simulink model "roach2_fengine_nlb"  (R2013b)
settings: Solver=VariableStepDiscrete  SolverMode=SingleTasking  StartTime=0.0  StopTime=10.0  RelTol=1e-3
undefined symbols (not defined in the file or in its folder): sfp
libraries: xbsIndex_r4 x3316, xps_library x74, casper_library_sources x16, casper_library_misc x7
(part 16 of 38)

== system roach2_fengine_nlb/eth/3/gbe_gpu_en ==
  in : Inport
  Logical : xbsIndex_r4/Logical  logical_function=AND  inputs=2  en=off  latency=1  precision=Full  arith_type=Unsigned  n_bits=16  bin_pt=0  align_bp=on  dbl_ovrd=off  block_type=logical
  out : Outport
  wires:
  [gbe_gpu_en] -> Logical/1
  Logical/1 -> out/1
  in/1 -> Logical/2

== system roach2_fengine_nlb/eth/3/gbe_sw_en ==
  in : Inport
  Logical : xbsIndex_r4/Logical  logical_function=AND  inputs=2  en=off  latency=0  precision=Full  arith_type=Unsigned  n_bits=16  bin_pt=0  align_bp=on  dbl_ovrd=off  block_type=logical
  out : Outport
  wires:
  in/1 -> Logical/2
  Logical/1 -> out/1
  [gbe_sw_en] -> Logical/1

== system roach2_fengine_nlb/eth/3/gpu_mon ==
  oflow : Inport
  Counter3 : xbsIndex_r4/Counter  cnt_type=Free Running  cnt_to=Inf  operation=Up  start_count=0  cnt_by_val=1  arith_type=Unsigned  n_bits=32  bin_pt=0  load_pin=off  rst=on  en=on  explicit_period=on  period=1  dbl_ovrd=off  use_behavioral_HDL=off  implementation=Fabric  block_type=counter
  Delay3 : xbsIndex_r4/Delay  rst=off  infoeditControl=Selection of Reset will increase slice count due to use of real FFs and instead of SRLs  en=off  latency=1  dbl_ovrd=off  reg_retiming=off  block_type=delay
  Delay6 : xbsIndex_r4/Delay  rst=off  infoeditControl=Selection of Reset will increase slice count due to use of real FFs and instead of SRLs  en=off  latency=1  dbl_ovrd=off  reg_retiming=off  block_type=delay
  oflow_cnt : Outport
  wires:
  Delay3/1 -> Counter3/2
  oflow/1 -> Delay3/1
  Delay6/1 -> oflow_cnt/1
  [cnt_rst] -> Counter3/1
  Counter3/1 -> Delay6/1

== system roach2_fengine_nlb/eth/3/sw_mon ==
  bfr : Inport
  orun : Inport  Port=2
  oflow : Inport  Port=3
  Counter1 : xbsIndex_r4/Counter  cnt_type=Free Running  cnt_to=Inf  operation=Up  start_count=0  cnt_by_val=1  arith_type=Unsigned  n_bits=32  bin_pt=0  load_pin=off  rst=on  en=on  explicit_period=on  period=1  dbl_ovrd=off  use_behavioral_HDL=off  implementation=Fabric  block_type=counter
  Counter2 : xbsIndex_r4/Counter  cnt_type=Free Running  cnt_to=Inf  operation=Up  start_count=0  cnt_by_val=1  arith_type=Unsigned  n_bits=32  bin_pt=0  load_pin=off  rst=on  en=on  explicit_period=on  period=1  dbl_ovrd=off  use_behavioral_HDL=off  implementation=Fabric  block_type=counter
  Counter3 : xbsIndex_r4/Counter  cnt_type=Free Running  cnt_to=Inf  operation=Up  start_count=0  cnt_by_val=1  arith_type=Unsigned  n_bits=32  bin_pt=0  load_pin=off  rst=on  en=on  explicit_period=on  period=1  dbl_ovrd=off  use_behavioral_HDL=off  implementation=Fabric  block_type=counter
  Delay{1..3,5..7} (6 alike) : xbsIndex_r4/Delay  rst=off  infoeditControl=Selection of Reset will increase slice count due to use of real FFs and instead of SRLs  en=off  latency=1  dbl_ovrd=off  reg_retiming=off  block_type=delay
  bfr_cnt : Outport
  orun_cnt : Outport  Port=2
  oflow_cnt : Outport  Port=3
  wires:
  Counter2/1 -> Delay5/1
  [cnt_rst] -> Counter2/1
  Counter1/1 -> Delay7/1
  [cnt_rst] -> Counter1/1
  Counter3/1 -> Delay6/1
  [cnt_rst] -> Counter3/1
  Delay5/1 -> bfr_cnt/1
  bfr/1 -> Delay1/1
  Delay7/1 -> orun_cnt/1
  orun/1 -> Delay2/1
  Delay6/1 -> oflow_cnt/1
  oflow/1 -> Delay3/1
  Delay1/1 -> Counter2/2
  Delay2/1 -> Counter1/2
  Delay3/1 -> Counter3/2

== system roach2_fengine_nlb/input/mux_0_31/in_snap ==
  In1 : Inport
  In2 : Inport  Port=2
  In3 : Inport  Port=3
  In4 : Inport  Port=4
  BitBasher : xbsIndex_r4/BitBasher  bitexpr=|  display_expr=off  sr_1=1  arith_type1=Unsigned  bin_pt1=0  sr_2=2  arith_type2=Unsigned  bin_pt2=0  sr_3=3  arith_type3=Unsigned  bin_pt3=0  sr_4=4  arith_type4=Unsigned  bin_pt4=0  dbl_ovrd=off  block_type=bitbasher
      | <!DOCTYPE HTML PUBLIC "-//W3C//DTD HTML 4.0//EN" "http://www.w3.org/TR/REC-html40/strict.dtd">
      | <html><head><meta name="qrichtext" content="1" /><style type="text/css">
      | p, li { white-space: pre-wrap; }
      | </style></head><body style=" font-family:'Sans'; font-size:10pt; font-weight:400; font-style:normal;">
      | <p style=" margin-top:12px; margin-bottom:12px; margin-left:0px; margin-right:0px; -qt-block-indent:0; text-indent:0px;"><span style=" font-family:'MS Shell Dlg'; font-size:8pt;">w32={d8,c8,b8,a8}</span></p></body></html>
  Delay : xbsIndex_r4/Delay  rst=off  infoeditControl=Selection of Reset will increase slice count due to use of real FFs and instead of SRLs  en=off  latency=3  dbl_ovrd=off  reg_retiming=on  block_type=delay
  tag scope: in_snap=global
  wires:
  BitBasher/1 -> Delay/1
  Delay/1 -> [in_snap]
  In1/1 -> BitBasher/1
  In2/1 -> BitBasher/2
  In3/1 -> BitBasher/3
  In4/1 -> BitBasher/4

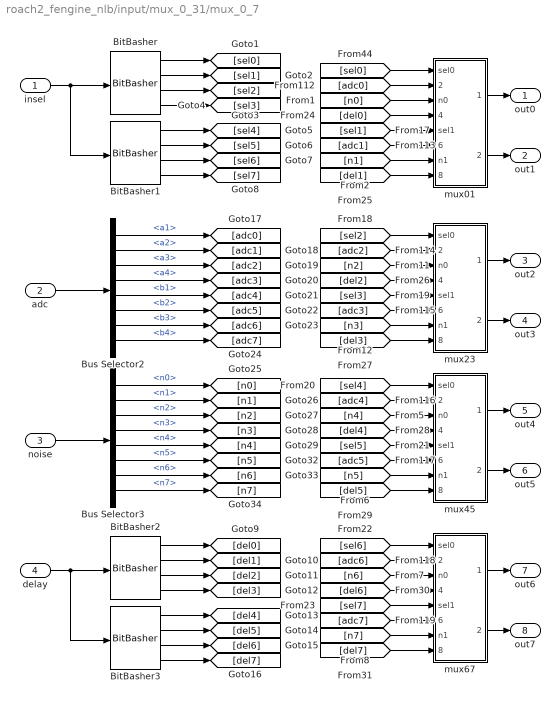
== system roach2_fengine_nlb/input/mux_0_31/mux_0_7 ==
  insel : Inport
  adc : Inport  Port=2
  noise : Inport  Port=3
  delay : Inport  Port=4
  BitBasher : xbsIndex_r4/BitBasher  bitexpr=|  display_expr=off  sr_1=1  arith_type1=Unsigned  bin_pt1=0  sr_2=2  arith_type2=Unsigned  bin_pt2=0  sr_3=3  arith_type3=Unsigned  bin_pt3=0  sr_4=4  arith_type4=Unsigned  bin_pt4=0  dbl_ovrd=off  block_type=bitbasher
      | <!DOCTYPE HTML PUBLIC "-//W3C//DTD HTML 4.0//EN" "http://www.w3.org/TR/REC-html40/strict.dtd">
      | <html><head><meta name="qrichtext" content="1" /><style type="text/css">
      | p, li { white-space: pre-wrap; }
      | </style></head><body style=" font-family:'Sans'; font-size:10pt; font-weight:400; font-style:normal;">
      | <p style=" margin-top:12px; margin-bottom:12px; margin-left:0px; margin-right:0px; -qt-block-indent:0; text-indent:0px;"><span style=" font-family:'MS Shell Dlg'; font-size:8pt;">s0={sel[1:0]}<br />s1={sel[5:4]}<br />s2={sel[9:8]}<br />s3={sel[13:12]}</span></p></body></html>
  BitBasher1 : xbsIndex_r4/BitBasher  bitexpr=|  display_expr=off  sr_1=1  arith_type1=Unsigned  bin_pt1=0  sr_2=2  arith_type2=Unsigned  bin_pt2=0  sr_3=3  arith_type3=Unsigned  bin_pt3=0  sr_4=4  arith_type4=Unsigned  bin_pt4=0  dbl_ovrd=off  block_type=bitbasher
      | <!DOCTYPE HTML PUBLIC "-//W3C//DTD HTML 4.0//EN" "http://www.w3.org/TR/REC-html40/strict.dtd">
      | <html><head><meta name="qrichtext" content="1" /><style type="text/css">
      | p, li { white-space: pre-wrap; }
      | </style></head><body style=" font-family:'Sans'; font-size:10pt; font-weight:400; font-style:normal;">
      | <p style=" margin-top:12px; margin-bottom:12px; margin-left:0px; margin-right:0px; -qt-block-indent:0; text-indent:0px;"><span style=" font-family:'MS Shell Dlg'; font-size:8pt;">s4={sel[17:16]}<br />s5={sel[21:20]}<br />s6={sel[25:24]}<br />s7={sel[29:28]}</span></p></body></html>
  BitBasher2 : xbsIndex_r4/BitBasher  bitexpr=|  display_expr=off  sr_1=1  arith_type1=Unsigned  bin_pt1=0  sr_2=2  arith_type2=Unsigned  bin_pt2=0  sr_3=3  arith_type3=Unsigned  bin_pt3=0  sr_4=4  arith_type4=Unsigned  bin_pt4=0  dbl_ovrd=off  block_type=bitbasher
      | <!DOCTYPE HTML PUBLIC "-//W3C//DTD HTML 4.0//EN" "http://www.w3.org/TR/REC-html40/strict.dtd">
      | <html><head><meta name="qrichtext" content="1" /><style type="text/css">
      | p, li { white-space: pre-wrap; }
      | </style></head><body style=" font-family:'Sans'; font-size:10pt; font-weight:400; font-style:normal;">
      | <p style=" margin-top:12px; margin-bottom:12px; margin-left:0px; margin-right:0px; -qt-block-indent:0; text-indent:0px;"><span style=" font-family:'MS Shell Dlg'; font-size:8pt;">d0={delay[7:0]}<br />d1={delay[15:8]}<br />d2={delay[23:16]}<br />d3={delay[31:24]}</span></p></body></html>
  BitBasher3 : xbsIndex_r4/BitBasher  bitexpr=|  display_expr=off  sr_1=1  arith_type1=Unsigned  bin_pt1=0  sr_2=2  arith_type2=Unsigned  bin_pt2=0  sr_3=3  arith_type3=Unsigned  bin_pt3=0  sr_4=4  arith_type4=Unsigned  bin_pt4=0  dbl_ovrd=off  block_type=bitbasher
      | <!DOCTYPE HTML PUBLIC "-//W3C//DTD HTML 4.0//EN" "http://www.w3.org/TR/REC-html40/strict.dtd">
      | <html><head><meta name="qrichtext" content="1" /><style type="text/css">
      | p, li { white-space: pre-wrap; }
      | </style></head><body style=" font-family:'Sans'; font-size:10pt; font-weight:400; font-style:normal;">
      | <p style=" margin-top:12px; margin-bottom:12px; margin-left:0px; margin-right:0px; -qt-block-indent:0; text-indent:0px;"><span style=" font-family:'MS Shell Dlg'; font-size:8pt;">d4={delay[39:32]}<br />d5={delay[47:40]}<br />d6={delay[55:48]}<br />d7={delay[63:56]}</span></p></body></html>
  Bus Selector2 : BusSelector  OutputSignals=a1,a2,a3,a4,b1,b2,b3,b4
  Bus Selector3 : BusSelector  OutputSignals=n0,n1,n2,n3,n4,n5,n6,n7
  mux01 : Subsystem
  mux23 : Subsystem
  mux45 : Subsystem
  mux67 : Subsystem
  out0 : Outport
  out1 : Outport  Port=2
  out2 : Outport  Port=3
  out3 : Outport  Port=4
  out4 : Outport  Port=5
  out5 : Outport  Port=6
  out6 : Outport  Port=7
  out7 : Outport  Port=8
  wires:
  [sel0] -> mux01/1(sel0)
  [adc0] -> mux01/2(adc0)
  [del0] -> mux01/4(delay0)
  [sel1] -> mux01/5(sel1)
  [adc1] -> mux01/6(adc1)
  [del1] -> mux01/8(delay1)
  BitBasher/1 -> [sel0]
  BitBasher/2 -> [sel1]
  BitBasher/3 -> [sel2]
  BitBasher/4 -> [sel3]
  BitBasher1/1 -> [sel4]
  BitBasher1/2 -> [sel5]
  BitBasher1/3 -> [sel6]
  BitBasher1/4 -> [sel7]
  [n0] -> mux01/3(n0)
  [n1] -> mux01/7(n1)
  [sel2] -> mux23/1(sel0)
  [adc2] -> mux23/2(adc0)
  [n2] -> mux23/3(n0)
  [del2] -> mux23/4(delay0)
  [sel3] -> mux23/5(sel1)
  [adc3] -> mux23/6(adc1)
  [n3] -> mux23/7(n1)
  [del3] -> mux23/8(delay1)
  [sel4] -> mux45/1(sel0)
  [adc4] -> mux45/2(adc0)
  [n4] -> mux45/3(n0)
  [del4] -> mux45/4(delay0)
  [sel5] -> mux45/5(sel1)
  [adc5] -> mux45/6(adc1)
  [n5] -> mux45/7(n1)
  [del5] -> mux45/8(delay1)
  [sel6] -> mux67/1(sel0)
  [adc6] -> mux67/2(adc0)
  [n6] -> mux67/3(n0)
  [del6] -> mux67/4(delay0)
  [sel7] -> mux67/5(sel1)
  [adc7] -> mux67/6(adc1)
  [n7] -> mux67/7(n1)
  [del7] -> mux67/8(delay1)
  insel/1 -> BitBasher1/1, BitBasher/1
  BitBasher2/1 -> [del0]
  BitBasher2/2 -> [del1]
  BitBasher2/3 -> [del2]
  BitBasher2/4 -> [del3]
  BitBasher3/1 -> [del4]
  BitBasher3/2 -> [del5]
  BitBasher3/3 -> [del6]
  BitBasher3/4 -> [del7]
  delay/1 -> BitBasher3/1, BitBasher2/1
  Bus Selector2/1 -> [adc0]  "<a1>"
  Bus Selector2/2 -> [adc1]  "<a2>"
  Bus Selector2/3 -> [adc2]  "<a3>"
  Bus Selector2/4 -> [adc3]  "<a4>"
  Bus Selector2/5 -> [adc4]  "<b1>"
  Bus Selector2/6 -> [adc5]  "<b2>"
  Bus Selector2/7 -> [adc6]  "<b3>"
  Bus Selector2/8 -> [adc7]  "<b4>"
  Bus Selector3/1 -> [n0]  "<n0>"
  Bus Selector3/2 -> [n1]  "<n1>"
  Bus Selector3/3 -> [n2]  "<n2>"
  Bus Selector3/4 -> [n3]  "<n3>"
  Bus Selector3/5 -> [n4]  "<n4>"
  Bus Selector3/6 -> [n5]  "<n5>"
  Bus Selector3/7 -> [n6]  "<n6>"
  Bus Selector3/8 -> [n7]  "<n7>"
  mux01/1(out0) -> out0/1
  mux01/2(out1) -> out1/1
  mux23/1(out0) -> out2/1
  adc/1 -> Bus Selector2/1
  mux23/2(out1) -> out3/1
  mux45/1(out0) -> out4/1
  noise/1 -> Bus Selector3/1
  mux45/2(out1) -> out5/1
  mux67/1(out0) -> out6/1
  mux67/2(out1) -> out7/1

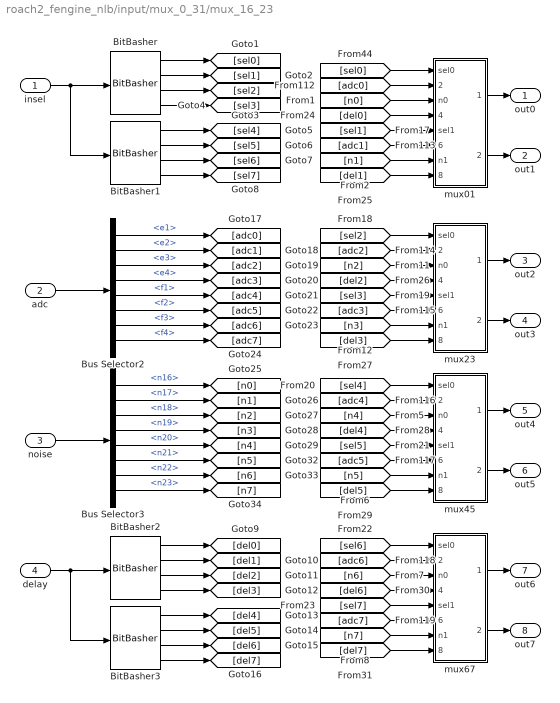
== system roach2_fengine_nlb/input/mux_0_31/mux_16_23 ==
  insel : Inport
  adc : Inport  Port=2
  noise : Inport  Port=3
  delay : Inport  Port=4
  BitBasher : xbsIndex_r4/BitBasher  bitexpr=|  display_expr=off  sr_1=1  arith_type1=Unsigned  bin_pt1=0  sr_2=2  arith_type2=Unsigned  bin_pt2=0  sr_3=3  arith_type3=Unsigned  bin_pt3=0  sr_4=4  arith_type4=Unsigned  bin_pt4=0  dbl_ovrd=off  block_type=bitbasher
      | <!DOCTYPE HTML PUBLIC "-//W3C//DTD HTML 4.0//EN" "http://www.w3.org/TR/REC-html40/strict.dtd">
      | <html><head><meta name="qrichtext" content="1" /><style type="text/css">
      | p, li { white-space: pre-wrap; }
      | </style></head><body style=" font-family:'Sans'; font-size:10pt; font-weight:400; font-style:normal;">
      | <p style=" margin-top:12px; margin-bottom:12px; margin-left:0px; margin-right:0px; -qt-block-indent:0; text-indent:0px;"><span style=" font-family:'MS Shell Dlg'; font-size:8pt;">s0={sel[1:0]}<br />s1={sel[5:4]}<br />s2={sel[9:8]}<br />s3={sel[13:12]}</span></p></body></html>
  BitBasher1 : xbsIndex_r4/BitBasher  bitexpr=|  display_expr=off  sr_1=1  arith_type1=Unsigned  bin_pt1=0  sr_2=2  arith_type2=Unsigned  bin_pt2=0  sr_3=3  arith_type3=Unsigned  bin_pt3=0  sr_4=4  arith_type4=Unsigned  bin_pt4=0  dbl_ovrd=off  block_type=bitbasher
      | <!DOCTYPE HTML PUBLIC "-//W3C//DTD HTML 4.0//EN" "http://www.w3.org/TR/REC-html40/strict.dtd">
      | <html><head><meta name="qrichtext" content="1" /><style type="text/css">
      | p, li { white-space: pre-wrap; }
      | </style></head><body style=" font-family:'Sans'; font-size:10pt; font-weight:400; font-style:normal;">
      | <p style=" margin-top:12px; margin-bottom:12px; margin-left:0px; margin-right:0px; -qt-block-indent:0; text-indent:0px;"><span style=" font-family:'MS Shell Dlg'; font-size:8pt;">s4={sel[17:16]}<br />s5={sel[21:20]}<br />s6={sel[25:24]}<br />s7={sel[29:28]}</span></p></body></html>
  BitBasher2 : xbsIndex_r4/BitBasher  bitexpr=|  display_expr=off  sr_1=1  arith_type1=Unsigned  bin_pt1=0  sr_2=2  arith_type2=Unsigned  bin_pt2=0  sr_3=3  arith_type3=Unsigned  bin_pt3=0  sr_4=4  arith_type4=Unsigned  bin_pt4=0  dbl_ovrd=off  block_type=bitbasher
      | <!DOCTYPE HTML PUBLIC "-//W3C//DTD HTML 4.0//EN" "http://www.w3.org/TR/REC-html40/strict.dtd">
      | <html><head><meta name="qrichtext" content="1" /><style type="text/css">
      | p, li { white-space: pre-wrap; }
      | </style></head><body style=" font-family:'Sans'; font-size:10pt; font-weight:400; font-style:normal;">
      | <p style=" margin-top:12px; margin-bottom:12px; margin-left:0px; margin-right:0px; -qt-block-indent:0; text-indent:0px;"><span style=" font-family:'MS Shell Dlg'; font-size:8pt;">d0={delay[7:0]}<br />d1={delay[15:8]}<br />d2={delay[23:16]}<br />d3={delay[31:24]}</span></p></body></html>
  BitBasher3 : xbsIndex_r4/BitBasher  bitexpr=|  display_expr=off  sr_1=1  arith_type1=Unsigned  bin_pt1=0  sr_2=2  arith_type2=Unsigned  bin_pt2=0  sr_3=3  arith_type3=Unsigned  bin_pt3=0  sr_4=4  arith_type4=Unsigned  bin_pt4=0  dbl_ovrd=off  block_type=bitbasher
      | <!DOCTYPE HTML PUBLIC "-//W3C//DTD HTML 4.0//EN" "http://www.w3.org/TR/REC-html40/strict.dtd">
      | <html><head><meta name="qrichtext" content="1" /><style type="text/css">
      | p, li { white-space: pre-wrap; }
      | </style></head><body style=" font-family:'Sans'; font-size:10pt; font-weight:400; font-style:normal;">
      | <p style=" margin-top:12px; margin-bottom:12px; margin-left:0px; margin-right:0px; -qt-block-indent:0; text-indent:0px;"><span style=" font-family:'MS Shell Dlg'; font-size:8pt;">d4={delay[39:32]}<br />d5={delay[47:40]}<br />d6={delay[55:48]}<br />d7={delay[63:56]}</span></p></body></html>
  Bus Selector2 : BusSelector  OutputSignals=e1,e2,e3,e4,f1,f2,f3,f4
  Bus Selector3 : BusSelector  OutputSignals=n16,n17,n18,n19,n20,n21,n22,n23
  mux01 : Subsystem
  mux23 : Subsystem
  mux45 : Subsystem
  mux67 : Subsystem
  out0 : Outport
  out1 : Outport  Port=2
  out2 : Outport  Port=3
  out3 : Outport  Port=4
  out4 : Outport  Port=5
  out5 : Outport  Port=6
  out6 : Outport  Port=7
  out7 : Outport  Port=8
  wires:
  mux67/2(out1) -> out7/1
  mux67/1(out0) -> out6/1
  mux45/2(out1) -> out5/1
  noise/1 -> Bus Selector3/1
  mux45/1(out0) -> out4/1
  mux23/2(out1) -> out3/1
  adc/1 -> Bus Selector2/1
  mux23/1(out0) -> out2/1
  mux01/2(out1) -> out1/1
  mux01/1(out0) -> out0/1
  Bus Selector3/8 -> [n7]  "<n23>"
  Bus Selector3/7 -> [n6]  "<n22>"
  Bus Selector3/6 -> [n5]  "<n21>"
  Bus Selector3/5 -> [n4]  "<n20>"
  Bus Selector3/4 -> [n3]  "<n19>"
  Bus Selector3/3 -> [n2]  "<n18>"
  Bus Selector3/2 -> [n1]  "<n17>"
  Bus Selector3/1 -> [n0]  "<n16>"
  Bus Selector2/8 -> [adc7]  "<f4>"
  Bus Selector2/7 -> [adc6]  "<f3>"
  Bus Selector2/6 -> [adc5]  "<f2>"
  Bus Selector2/5 -> [adc4]  "<f1>"
  Bus Selector2/4 -> [adc3]  "<e4>"
  Bus Selector2/3 -> [adc2]  "<e3>"
  Bus Selector2/2 -> [adc1]  "<e2>"
  Bus Selector2/1 -> [adc0]  "<e1>"
  delay/1 -> BitBasher2/1, BitBasher3/1
  BitBasher3/4 -> [del7]
  BitBasher3/3 -> [del6]
  BitBasher3/2 -> [del5]
  BitBasher3/1 -> [del4]
  BitBasher2/4 -> [del3]
  BitBasher2/3 -> [del2]
  BitBasher2/2 -> [del1]
  BitBasher2/1 -> [del0]
  insel/1 -> BitBasher/1, BitBasher1/1
  [del7] -> mux67/8(delay1)
  [n7] -> mux67/7(n1)
  [adc7] -> mux67/6(adc1)
  [sel7] -> mux67/5(sel1)
  [del6] -> mux67/4(delay0)
  [n6] -> mux67/3(n0)
  [adc6] -> mux67/2(adc0)
  [sel6] -> mux67/1(sel0)
  [del5] -> mux45/8(delay1)
  [n5] -> mux45/7(n1)
  [adc5] -> mux45/6(adc1)
  [sel5] -> mux45/5(sel1)
  [del4] -> mux45/4(delay0)
  [n4] -> mux45/3(n0)
  [adc4] -> mux45/2(adc0)
  [sel4] -> mux45/1(sel0)
  [del3] -> mux23/8(delay1)
  [n3] -> mux23/7(n1)
  [adc3] -> mux23/6(adc1)
  [sel3] -> mux23/5(sel1)
  [del2] -> mux23/4(delay0)
  [n2] -> mux23/3(n0)
  [adc2] -> mux23/2(adc0)
  [sel2] -> mux23/1(sel0)
  [n1] -> mux01/7(n1)
  [n0] -> mux01/3(n0)
  BitBasher1/4 -> [sel7]
  BitBasher1/3 -> [sel6]
  BitBasher1/2 -> [sel5]
  BitBasher1/1 -> [sel4]
  BitBasher/4 -> [sel3]
  BitBasher/3 -> [sel2]
  BitBasher/2 -> [sel1]
  BitBasher/1 -> [sel0]
  [del1] -> mux01/8(delay1)
  [adc1] -> mux01/6(adc1)
  [sel1] -> mux01/5(sel1)
  [del0] -> mux01/4(delay0)
  [adc0] -> mux01/2(adc0)
  [sel0] -> mux01/1(sel0)

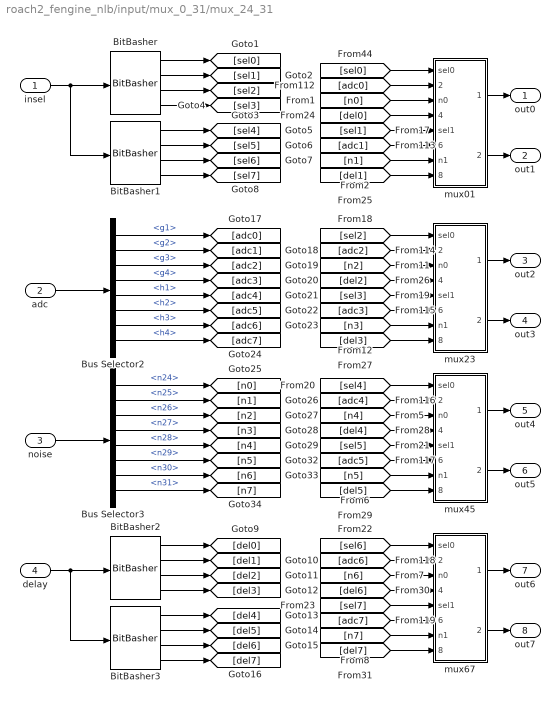
== system roach2_fengine_nlb/input/mux_0_31/mux_24_31 ==
  insel : Inport
  adc : Inport  Port=2
  noise : Inport  Port=3
  delay : Inport  Port=4
  BitBasher : xbsIndex_r4/BitBasher  bitexpr=|  display_expr=off  sr_1=1  arith_type1=Unsigned  bin_pt1=0  sr_2=2  arith_type2=Unsigned  bin_pt2=0  sr_3=3  arith_type3=Unsigned  bin_pt3=0  sr_4=4  arith_type4=Unsigned  bin_pt4=0  dbl_ovrd=off  block_type=bitbasher
      | <!DOCTYPE HTML PUBLIC "-//W3C//DTD HTML 4.0//EN" "http://www.w3.org/TR/REC-html40/strict.dtd">
      | <html><head><meta name="qrichtext" content="1" /><style type="text/css">
      | p, li { white-space: pre-wrap; }
      | </style></head><body style=" font-family:'Sans'; font-size:10pt; font-weight:400; font-style:normal;">
      | <p style=" margin-top:12px; margin-bottom:12px; margin-left:0px; margin-right:0px; -qt-block-indent:0; text-indent:0px;"><span style=" font-family:'MS Shell Dlg'; font-size:8pt;">s0={sel[1:0]}<br />s1={sel[5:4]}<br />s2={sel[9:8]}<br />s3={sel[13:12]}</span></p></body></html>
  BitBasher1 : xbsIndex_r4/BitBasher  bitexpr=|  display_expr=off  sr_1=1  arith_type1=Unsigned  bin_pt1=0  sr_2=2  arith_type2=Unsigned  bin_pt2=0  sr_3=3  arith_type3=Unsigned  bin_pt3=0  sr_4=4  arith_type4=Unsigned  bin_pt4=0  dbl_ovrd=off  block_type=bitbasher
      | <!DOCTYPE HTML PUBLIC "-//W3C//DTD HTML 4.0//EN" "http://www.w3.org/TR/REC-html40/strict.dtd">
      | <html><head><meta name="qrichtext" content="1" /><style type="text/css">
      | p, li { white-space: pre-wrap; }
      | </style></head><body style=" font-family:'Sans'; font-size:10pt; font-weight:400; font-style:normal;">
      | <p style=" margin-top:12px; margin-bottom:12px; margin-left:0px; margin-right:0px; -qt-block-indent:0; text-indent:0px;"><span style=" font-family:'MS Shell Dlg'; font-size:8pt;">s4={sel[17:16]}<br />s5={sel[21:20]}<br />s6={sel[25:24]}<br />s7={sel[29:28]}</span></p></body></html>
  BitBasher2 : xbsIndex_r4/BitBasher  bitexpr=|  display_expr=off  sr_1=1  arith_type1=Unsigned  bin_pt1=0  sr_2=2  arith_type2=Unsigned  bin_pt2=0  sr_3=3  arith_type3=Unsigned  bin_pt3=0  sr_4=4  arith_type4=Unsigned  bin_pt4=0  dbl_ovrd=off  block_type=bitbasher
      | <!DOCTYPE HTML PUBLIC "-//W3C//DTD HTML 4.0//EN" "http://www.w3.org/TR/REC-html40/strict.dtd">
      | <html><head><meta name="qrichtext" content="1" /><style type="text/css">
      | p, li { white-space: pre-wrap; }
      | </style></head><body style=" font-family:'Sans'; font-size:10pt; font-weight:400; font-style:normal;">
      | <p style=" margin-top:12px; margin-bottom:12px; margin-left:0px; margin-right:0px; -qt-block-indent:0; text-indent:0px;"><span style=" font-family:'MS Shell Dlg'; font-size:8pt;">d0={delay[7:0]}<br />d1={delay[15:8]}<br />d2={delay[23:16]}<br />d3={delay[31:24]}</span></p></body></html>
  BitBasher3 : xbsIndex_r4/BitBasher  bitexpr=|  display_expr=off  sr_1=1  arith_type1=Unsigned  bin_pt1=0  sr_2=2  arith_type2=Unsigned  bin_pt2=0  sr_3=3  arith_type3=Unsigned  bin_pt3=0  sr_4=4  arith_type4=Unsigned  bin_pt4=0  dbl_ovrd=off  block_type=bitbasher
      | <!DOCTYPE HTML PUBLIC "-//W3C//DTD HTML 4.0//EN" "http://www.w3.org/TR/REC-html40/strict.dtd">
      | <html><head><meta name="qrichtext" content="1" /><style type="text/css">
      | p, li { white-space: pre-wrap; }
      | </style></head><body style=" font-family:'Sans'; font-size:10pt; font-weight:400; font-style:normal;">
      | <p style=" margin-top:12px; margin-bottom:12px; margin-left:0px; margin-right:0px; -qt-block-indent:0; text-indent:0px;"><span style=" font-family:'MS Shell Dlg'; font-size:8pt;">d4={delay[39:32]}<br />d5={delay[47:40]}<br />d6={delay[55:48]}<br />d7={delay[63:56]}</span></p></body></html>
  Bus Selector2 : BusSelector  OutputSignals=g1,g2,g3,g4,h1,h2,h3,h4
  Bus Selector3 : BusSelector  OutputSignals=n24,n25,n26,n27,n28,n29,n30,n31
  mux01 : Subsystem
  mux23 : Subsystem
  mux45 : Subsystem
  mux67 : Subsystem
  out0 : Outport
  out1 : Outport  Port=2
  out2 : Outport  Port=3
  out3 : Outport  Port=4
  out4 : Outport  Port=5
  out5 : Outport  Port=6
  out6 : Outport  Port=7
  out7 : Outport  Port=8
  wires:
  [sel0] -> mux01/1(sel0)
  [adc0] -> mux01/2(adc0)
  [del0] -> mux01/4(delay0)
  [sel1] -> mux01/5(sel1)
  [adc1] -> mux01/6(adc1)
  [del1] -> mux01/8(delay1)
  BitBasher/1 -> [sel0]
  BitBasher/2 -> [sel1]
  BitBasher/3 -> [sel2]
  BitBasher/4 -> [sel3]
  BitBasher1/1 -> [sel4]
  BitBasher1/2 -> [sel5]
  BitBasher1/3 -> [sel6]
  BitBasher1/4 -> [sel7]
  [n0] -> mux01/3(n0)
  [n1] -> mux01/7(n1)
  [sel2] -> mux23/1(sel0)
  [adc2] -> mux23/2(adc0)
  [n2] -> mux23/3(n0)
  [del2] -> mux23/4(delay0)
  [sel3] -> mux23/5(sel1)
  [adc3] -> mux23/6(adc1)
  [n3] -> mux23/7(n1)
  [del3] -> mux23/8(delay1)
  [sel4] -> mux45/1(sel0)
  [adc4] -> mux45/2(adc0)
  [n4] -> mux45/3(n0)
  [del4] -> mux45/4(delay0)
  [sel5] -> mux45/5(sel1)
  [adc5] -> mux45/6(adc1)
  [n5] -> mux45/7(n1)
  [del5] -> mux45/8(delay1)
  [sel6] -> mux67/1(sel0)
  [adc6] -> mux67/2(adc0)
  [n6] -> mux67/3(n0)
  [del6] -> mux67/4(delay0)
  [sel7] -> mux67/5(sel1)
  [adc7] -> mux67/6(adc1)
  [n7] -> mux67/7(n1)
  [del7] -> mux67/8(delay1)
  insel/1 -> BitBasher1/1, BitBasher/1
  BitBasher2/1 -> [del0]
  BitBasher2/2 -> [del1]
  BitBasher2/3 -> [del2]
  BitBasher2/4 -> [del3]
  BitBasher3/1 -> [del4]
  BitBasher3/2 -> [del5]
  BitBasher3/3 -> [del6]
  BitBasher3/4 -> [del7]
  delay/1 -> BitBasher3/1, BitBasher2/1
  Bus Selector2/1 -> [adc0]  "<g1>"
  Bus Selector2/2 -> [adc1]  "<g2>"
  Bus Selector2/3 -> [adc2]  "<g3>"
  Bus Selector2/4 -> [adc3]  "<g4>"
  Bus Selector2/5 -> [adc4]  "<h1>"
  Bus Selector2/6 -> [adc5]  "<h2>"
  Bus Selector2/7 -> [adc6]  "<h3>"
  Bus Selector2/8 -> [adc7]  "<h4>"
  Bus Selector3/1 -> [n0]  "<n24>"
  Bus Selector3/2 -> [n1]  "<n25>"
  Bus Selector3/3 -> [n2]  "<n26>"
  Bus Selector3/4 -> [n3]  "<n27>"
  Bus Selector3/5 -> [n4]  "<n28>"
  Bus Selector3/6 -> [n5]  "<n29>"
  Bus Selector3/7 -> [n6]  "<n30>"
  Bus Selector3/8 -> [n7]  "<n31>"
  mux01/1(out0) -> out0/1
  mux01/2(out1) -> out1/1
  mux23/1(out0) -> out2/1
  adc/1 -> Bus Selector2/1
  mux23/2(out1) -> out3/1
  mux45/1(out0) -> out4/1
  noise/1 -> Bus Selector3/1
  mux45/2(out1) -> out5/1
  mux67/1(out0) -> out6/1
  mux67/2(out1) -> out7/1

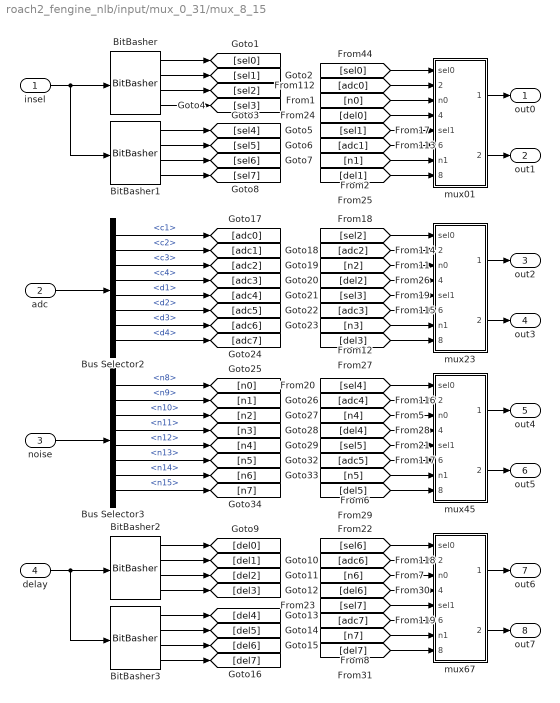
== system roach2_fengine_nlb/input/mux_0_31/mux_8_15 ==
  insel : Inport
  adc : Inport  Port=2
  noise : Inport  Port=3
  delay : Inport  Port=4
  BitBasher : xbsIndex_r4/BitBasher  bitexpr=|  display_expr=off  sr_1=1  arith_type1=Unsigned  bin_pt1=0  sr_2=2  arith_type2=Unsigned  bin_pt2=0  sr_3=3  arith_type3=Unsigned  bin_pt3=0  sr_4=4  arith_type4=Unsigned  bin_pt4=0  dbl_ovrd=off  block_type=bitbasher
      | <!DOCTYPE HTML PUBLIC "-//W3C//DTD HTML 4.0//EN" "http://www.w3.org/TR/REC-html40/strict.dtd">
      | <html><head><meta name="qrichtext" content="1" /><style type="text/css">
      | p, li { white-space: pre-wrap; }
      | </style></head><body style=" font-family:'Sans'; font-size:10pt; font-weight:400; font-style:normal;">
      | <p style=" margin-top:12px; margin-bottom:12px; margin-left:0px; margin-right:0px; -qt-block-indent:0; text-indent:0px;"><span style=" font-family:'MS Shell Dlg'; font-size:8pt;">s0={sel[1:0]}<br />s1={sel[5:4]}<br />s2={sel[9:8]}<br />s3={sel[13:12]}</span></p></body></html>
  BitBasher1 : xbsIndex_r4/BitBasher  bitexpr=|  display_expr=off  sr_1=1  arith_type1=Unsigned  bin_pt1=0  sr_2=2  arith_type2=Unsigned  bin_pt2=0  sr_3=3  arith_type3=Unsigned  bin_pt3=0  sr_4=4  arith_type4=Unsigned  bin_pt4=0  dbl_ovrd=off  block_type=bitbasher
      | <!DOCTYPE HTML PUBLIC "-//W3C//DTD HTML 4.0//EN" "http://www.w3.org/TR/REC-html40/strict.dtd">
      | <html><head><meta name="qrichtext" content="1" /><style type="text/css">
      | p, li { white-space: pre-wrap; }
      | </style></head><body style=" font-family:'Sans'; font-size:10pt; font-weight:400; font-style:normal;">
      | <p style=" margin-top:12px; margin-bottom:12px; margin-left:0px; margin-right:0px; -qt-block-indent:0; text-indent:0px;"><span style=" font-family:'MS Shell Dlg'; font-size:8pt;">s4={sel[17:16]}<br />s5={sel[21:20]}<br />s6={sel[25:24]}<br />s7={sel[29:28]}</span></p></body></html>
  BitBasher2 : xbsIndex_r4/BitBasher  bitexpr=|  display_expr=off  sr_1=1  arith_type1=Unsigned  bin_pt1=0  sr_2=2  arith_type2=Unsigned  bin_pt2=0  sr_3=3  arith_type3=Unsigned  bin_pt3=0  sr_4=4  arith_type4=Unsigned  bin_pt4=0  dbl_ovrd=off  block_type=bitbasher
      | <!DOCTYPE HTML PUBLIC "-//W3C//DTD HTML 4.0//EN" "http://www.w3.org/TR/REC-html40/strict.dtd">
      | <html><head><meta name="qrichtext" content="1" /><style type="text/css">
      | p, li { white-space: pre-wrap; }
      | </style></head><body style=" font-family:'Sans'; font-size:10pt; font-weight:400; font-style:normal;">
      | <p style=" margin-top:12px; margin-bottom:12px; margin-left:0px; margin-right:0px; -qt-block-indent:0; text-indent:0px;"><span style=" font-family:'MS Shell Dlg'; font-size:8pt;">d0={delay[7:0]}<br />d1={delay[15:8]}<br />d2={delay[23:16]}<br />d3={delay[31:24]}</span></p></body></html>
  BitBasher3 : xbsIndex_r4/BitBasher  bitexpr=|  display_expr=off  sr_1=1  arith_type1=Unsigned  bin_pt1=0  sr_2=2  arith_type2=Unsigned  bin_pt2=0  sr_3=3  arith_type3=Unsigned  bin_pt3=0  sr_4=4  arith_type4=Unsigned  bin_pt4=0  dbl_ovrd=off  block_type=bitbasher
      | <!DOCTYPE HTML PUBLIC "-//W3C//DTD HTML 4.0//EN" "http://www.w3.org/TR/REC-html40/strict.dtd">
      | <html><head><meta name="qrichtext" content="1" /><style type="text/css">
      | p, li { white-space: pre-wrap; }
      | </style></head><body style=" font-family:'Sans'; font-size:10pt; font-weight:400; font-style:normal;">
      | <p style=" margin-top:12px; margin-bottom:12px; margin-left:0px; margin-right:0px; -qt-block-indent:0; text-indent:0px;"><span style=" font-family:'MS Shell Dlg'; font-size:8pt;">d4={delay[39:32]}<br />d5={delay[47:40]}<br />d6={delay[55:48]}<br />d7={delay[63:56]}</span></p></body></html>
  Bus Selector2 : BusSelector  OutputSignals=c1,c2,c3,c4,d1,d2,d3,d4
  Bus Selector3 : BusSelector  OutputSignals=n8,n9,n10,n11,n12,n13,n14,n15
  mux01 : Subsystem
  mux23 : Subsystem
  mux45 : Subsystem
  mux67 : Subsystem
  out0 : Outport
  out1 : Outport  Port=2
  out2 : Outport  Port=3
  out3 : Outport  Port=4
  out4 : Outport  Port=5
  out5 : Outport  Port=6
  out6 : Outport  Port=7
  out7 : Outport  Port=8
  wires:
  mux67/2(out1) -> out7/1
  mux67/1(out0) -> out6/1
  mux45/2(out1) -> out5/1
  noise/1 -> Bus Selector3/1
  mux45/1(out0) -> out4/1
  mux23/2(out1) -> out3/1
  adc/1 -> Bus Selector2/1
  mux23/1(out0) -> out2/1
  mux01/2(out1) -> out1/1
  mux01/1(out0) -> out0/1
  Bus Selector3/8 -> [n7]  "<n15>"
  Bus Selector3/7 -> [n6]  "<n14>"
  Bus Selector3/6 -> [n5]  "<n13>"
  Bus Selector3/5 -> [n4]  "<n12>"
  Bus Selector3/4 -> [n3]  "<n11>"
  Bus Selector3/3 -> [n2]  "<n10>"
  Bus Selector3/2 -> [n1]  "<n9>"
  Bus Selector3/1 -> [n0]  "<n8>"
  Bus Selector2/8 -> [adc7]  "<d4>"
  Bus Selector2/7 -> [adc6]  "<d3>"
  Bus Selector2/6 -> [adc5]  "<d2>"
  Bus Selector2/5 -> [adc4]  "<d1>"
  Bus Selector2/4 -> [adc3]  "<c4>"
  Bus Selector2/3 -> [adc2]  "<c3>"
  Bus Selector2/2 -> [adc1]  "<c2>"
  Bus Selector2/1 -> [adc0]  "<c1>"
  delay/1 -> BitBasher2/1, BitBasher3/1
  BitBasher3/4 -> [del7]
  BitBasher3/3 -> [del6]
  BitBasher3/2 -> [del5]
  BitBasher3/1 -> [del4]
  BitBasher2/4 -> [del3]
  BitBasher2/3 -> [del2]
  BitBasher2/2 -> [del1]
  BitBasher2/1 -> [del0]
  insel/1 -> BitBasher/1, BitBasher1/1
  [del7] -> mux67/8(delay1)
  [n7] -> mux67/7(n1)
  [adc7] -> mux67/6(adc1)
  [sel7] -> mux67/5(sel1)
  [del6] -> mux67/4(delay0)
  [n6] -> mux67/3(n0)
  [adc6] -> mux67/2(adc0)
  [sel6] -> mux67/1(sel0)
  [del5] -> mux45/8(delay1)
  [n5] -> mux45/7(n1)
  [adc5] -> mux45/6(adc1)
  [sel5] -> mux45/5(sel1)
  [del4] -> mux45/4(delay0)
  [n4] -> mux45/3(n0)
  [adc4] -> mux45/2(adc0)
  [sel4] -> mux45/1(sel0)
  [del3] -> mux23/8(delay1)
  [n3] -> mux23/7(n1)
  [adc3] -> mux23/6(adc1)
  [sel3] -> mux23/5(sel1)
  [del2] -> mux23/4(delay0)
  [n2] -> mux23/3(n0)
  [adc2] -> mux23/2(adc0)
  [sel2] -> mux23/1(sel0)
  [n1] -> mux01/7(n1)
  [n0] -> mux01/3(n0)
  BitBasher1/4 -> [sel7]
  BitBasher1/3 -> [sel6]
  BitBasher1/2 -> [sel5]
  BitBasher1/1 -> [sel4]
  BitBasher/4 -> [sel3]
  BitBasher/3 -> [sel2]
  BitBasher/2 -> [sel1]
  BitBasher/1 -> [sel0]
  [del1] -> mux01/8(delay1)
  [adc1] -> mux01/6(adc1)
  [sel1] -> mux01/5(sel1)
  [del0] -> mux01/4(delay0)
  [adc0] -> mux01/2(adc0)
  [sel0] -> mux01/1(sel0)

== system roach2_fengine_nlb/input/rms/bram_ctrl ==
  adc0 : Inport
  adc1 : Inport  Port=2
  adc2 : Inport  Port=3
  adc3 : Inport  Port=4
  adc4 : Inport  Port=5
  adc5 : Inport  Port=6
  adc6 : Inport  Port=7
  adc7 : Inport  Port=8
  adc8 : Inport  Port=9
  adc9 : Inport  Port=10
  adc10 : Inport  Port=11
  adc11 : Inport  Port=12
  adc12 : Inport  Port=13
  adc13 : Inport  Port=14
  adc14 : Inport  Port=15
  adc15 : Inport  Port=16
  adc16 : Inport  Port=17
  adc17 : Inport  Port=18
  adc18 : Inport  Port=19
  adc19 : Inport  Port=20
  adc20 : Inport  Port=21
  adc21 : Inport  Port=22
  adc22 : Inport  Port=23
  adc23 : Inport  Port=24
  adc24 : Inport  Port=25
  adc25 : Inport  Port=26
  adc26 : Inport  Port=27
  adc27 : Inport  Port=28
  adc28 : Inport  Port=29
  adc29 : Inport  Port=30
  adc30 : Inport  Port=31
  adc31 : Inport  Port=32
  en : Inport  Port=33
  BitBasher : xbsIndex_r4/BitBasher  bitexpr=|  display_expr=off  sr_1=1  arith_type1="Signed  (2's comp)"  bin_pt1=0  sr_2=2  arith_type2=Unsigned  bin_pt2=0  sr_3=3  arith_type3=Unsigned  bin_pt3=0  sr_4=4  arith_type4=Unsigned  bin_pt4=0  dbl_ovrd=off  block_type=bitbasher
      | <!DOCTYPE HTML PUBLIC "-//W3C//DTD HTML 4.0//EN" "http://www.w3.org/TR/REC-html40/strict.dtd">
      | <html><head><meta name="qrichtext" content="1" /><style type="text/css">
      | p, li { white-space: pre-wrap; }
      | </style></head><body style=" font-family:'Sans'; font-size:10pt; font-weight:400; font-style:normal;">
      | <p style=" margin-top:12px; margin-bottom:12px; margin-left:0px; margin-right:0px; -qt-block-indent:0; text-indent:0px;"><span style=" font-family:'MS Shell Dlg'; font-size:8pt;">s={sss[55:32]}<br />ss={sss[31:0]}</span></p></body></html>
  Constant : xbsIndex_r4/Constant  const=1  gui_display_data_type=Boolean  arith_type=Boolean  n_bits=16  bin_pt=14  preci_type=Single  exp_width=8  frac_width=24  explicit_period=on  period=1  equ=P=C  opselect=C  inp2=PCIN>>17  opr=+  inp1=P  carry=CIN  dbl_ovrd=off  block_type=constant
  Convert2 : xbsIndex_r4/Convert  gui_display_data_type=Fixed-point  arith_type=Unsigned  n_bits=32  bin_pt=0  float_type=Single  exp_bits=8  fraction_bits=24  quantization=Truncate  overflow=Wrap  en=off  latency=0  dbl_ovrd=off  pipeline=off  block_type=convert
      settings: block_version=11.4
  Delay{1..5} (5 alike) : xbsIndex_r4/Delay  rst=off  infoeditControl=Selection of Reset will increase slice count due to use of real FFs and instead of SRLs  en=off  latency=1  dbl_ovrd=off  reg_retiming=off  block_type=delay
  Logical : xbsIndex_r4/Logical  logical_function=AND  inputs=2  en=off  latency=0  precision=Full  arith_type=Unsigned  n_bits=16  bin_pt=0  align_bp=on  dbl_ovrd=off  block_type=logical
  Mux : xbsIndex_r4/Mux  inputs=32  en=off  latency=1  precision=Full  arith_type=Unsigned  n_bits=16  bin_pt=14  quantization=Truncate  overflow=Wrap  dbl_ovrd=off  block_type=mux
  Mux1 : xbsIndex_r4/Mux  inputs=2  en=off  latency=1  precision=Full  arith_type=Unsigned  n_bits=16  bin_pt=14  quantization=Truncate  overflow=Wrap  dbl_ovrd=off  block_type=mux
  Slice3 : xbsIndex_r4/Slice  nbits=5  boolean_output=off  mode=Upper Bit Location + Width  bit1=0  base1=MSB of Input  bit0=19  base0=LSB of Input  dbl_ovrd=off  block_type=slice
      settings: block_version=10.1.3
  Slice6 : xbsIndex_r4/Slice  nbits=1  boolean_output=off  mode=Lower Bit Location + Width  bit1=0  base1=MSB of Input  bit0=0  base0=LSB of Input  dbl_ovrd=off  block_type=slice
      settings: block_version=10.1.3
  Terminator : Terminator
  freeze_cntr : casper_library_misc/freeze_cntr  CounterBits=6
  sign_extend : xbsIndex_r4/Convert  gui_display_data_type=Fixed-point  arith_type="Signed  (2's comp)"  n_bits=32  bin_pt=0  float_type=Single  exp_bits=8  fraction_bits=24  quantization=Truncate  overflow=Wrap  en=off  latency=0  dbl_ovrd=off  pipeline=off  block_type=convert
      settings: block_version=11.4
  addr : Outport
  data : Outport  Port=2
  we : Outport  Port=3
  wires:
  freeze_cntr/1 -> Slice3/1, Delay2/1
  Slice3/1 -> Mux/1
  adc0/1 -> Mux/2
  adc1/1 -> Mux/3
  adc2/1 -> Mux/4
  adc3/1 -> Mux/5
  Mux/1 -> BitBasher/1
  Mux1/1 -> data/1
  BitBasher/2 -> Delay1/1
  BitBasher/1 -> sign_extend/1
  Delay1/1 -> Mux1/3
  Logical/1 -> freeze_cntr/2
  [adc_rms_rst] -> Logical/1
  en/1 -> Logical/2
  freeze_cntr/2 -> Delay3/1
  Slice6/1 -> Mux1/1
  Constant/1 -> freeze_cntr/1
  adc4/1 -> Mux/6
  adc5/1 -> Mux/7
  adc6/1 -> Mux/8
  adc7/1 -> Mux/9
  adc8/1 -> Mux/10
  adc9/1 -> Mux/11
  adc10/1 -> Mux/12
  adc11/1 -> Mux/13
  adc12/1 -> Mux/14
  adc13/1 -> Mux/15
  adc14/1 -> Mux/16
  adc15/1 -> Mux/17
  adc16/1 -> Mux/18
  adc17/1 -> Mux/19
  adc18/1 -> Mux/20
  adc19/1 -> Mux/21
  adc20/1 -> Mux/22
  adc21/1 -> Mux/23
  adc22/1 -> Mux/24
  adc23/1 -> Mux/25
  adc24/1 -> Mux/26
  adc25/1 -> Mux/27
  adc26/1 -> Mux/28
  adc27/1 -> Mux/29
  adc28/1 -> Mux/30
  adc29/1 -> Mux/31
  adc30/1 -> Mux/32
  adc31/1 -> Mux/33
  Delay2/1 -> Slice6/1, Delay4/1
  Delay3/1 -> Delay5/1
  Delay4/1 -> addr/1
  Delay5/1 -> we/1
  Convert2/1 -> Mux1/2
  freeze_cntr/3 -> Terminator/1
  sign_extend/1 -> Convert2/1

== system roach2_fengine_nlb/input/rms/calc_adc_sum_sq0 ==
  note: 127^2 == 16129
  in : Inport
  Accumulator : xbsIndex_r4/Accumulator  operation=Add  n_bits=32  overflow=Wrap  scale=1  rst=on  infoeditControl=reset for floating point data type must be asserted for a minimum of 2 cycles  hasbypass=on  en=off  latency=0  dbl_ovrd=off  msb_inp=100  msb=100  lsb=-100  use_behavioral_HDL=on  implementation=Fabric  block_type=accum
      settings: infoedit="Adder or subtractor-based accumulator.   Output type and binary point position match the input.<P><P>Hardware notes: When \"Reinitialize with input 'b' on reset\" is selected, the accumulator is forced to run at the system rate even if the input 'b' is running at a slower rate."  xl_area=[0, 0, 0, 0, 0, 0, 0]  block_version=10.1.3
  Accumulator1 : xbsIndex_r4/Accumulator  operation=Add  n_bits=24  overflow=Wrap  scale=1  rst=on  infoeditControl=reset for floating point data type must be asserted for a minimum of 2 cycles  hasbypass=on  en=off  latency=0  dbl_ovrd=off  msb_inp=100  msb=100  lsb=-100  use_behavioral_HDL=on  implementation=Fabric  block_type=accum
      settings: infoedit="Adder or subtractor-based accumulator.   Output type and binary point position match the input.<P><P>Hardware notes: When \"Reinitialize with input 'b' on reset\" is selected, the accumulator is forced to run at the system rate even if the input 'b' is running at a slower rate."  xl_area=[0, 0, 0, 0, 0, 0, 0]  block_version=10.1.3
  BitBasher : xbsIndex_r4/BitBasher  bitexpr=|  display_expr=off  sr_1=1  arith_type1="Signed  (2's comp)"  bin_pt1=0  sr_2=2  arith_type2=Unsigned  bin_pt2=0  sr_3=3  arith_type3=Unsigned  bin_pt3=0  sr_4=4  arith_type4=Unsigned  bin_pt4=0  dbl_ovrd=off  block_type=bitbasher
      | <!DOCTYPE HTML PUBLIC "-//W3C//DTD HTML 4.0//EN" "http://www.w3.org/TR/REC-html40/strict.dtd">
      | <html><head><meta name="qrichtext" content="1" /><style type="text/css">
      | p, li { white-space: pre-wrap; }
      | </style></head><body style=" font-family:'Sans'; font-size:10pt; font-weight:400; font-style:normal;">
      | <p style=" margin-top:12px; margin-bottom:12px; margin-left:0px; margin-right:0px; -qt-block-indent:0; text-indent:0px;"><span style=" font-family:'MS Shell Dlg'; font-size:8pt;">sss={s,ss}</span></p></body></html>
      settings: block_version=10.1.3
  Constant : xbsIndex_r4/Constant  const=127^2  gui_display_data_type=Fixed-point  arith_type=Unsigned  n_bits=15  bin_pt=0  preci_type=Single  exp_width=8  frac_width=24  explicit_period=on  period=1  equ=P=C  opselect=C  inp2=PCIN>>17  opr=+  inp1=P  carry=CIN  dbl_ovrd=off  block_type=constant
  Delay : xbsIndex_r4/Delay  rst=off  infoeditControl=Selection of Reset will increase slice count due to use of real FFs and instead of SRLs  en=off  latency=2  dbl_ovrd=off  reg_retiming=off  block_type=delay
  Delay1 : xbsIndex_r4/Delay  rst=off  infoeditControl=Selection of Reset will increase slice count due to use of real FFs and instead of SRLs  en=off  latency=1  dbl_ovrd=off  reg_retiming=off  block_type=delay
  Mult : xbsIndex_r4/Mult  precision=User Defined  arith_type=Unsigned  n_bits=15  bin_pt=0  quantization=Truncate  overflow=Wrap  en=off  latency=2  dbl_ovrd=off  use_behavioral_HDL=on  opt=Speed  use_embedded=on  optimum_pipeline=on  pipeline=on  use_rpm=on  placement_style=Rectangular shape  block_type=mult
      settings: xl_area=[0, 0, 0, 0, 0, 0, 0]  block_version=10.1.3
  Register : xbsIndex_r4/Register  init=0  rst=off  en=on  dbl_ovrd=off  block_type=register
      settings: xl_area=[0, 0, 0, 0, 0, 0, 0]
  Register1 : xbsIndex_r4/Register  init=0  rst=off  en=on  dbl_ovrd=off  block_type=register
      settings: xl_area=[0, 0, 0, 0, 0, 0, 0]
  Reinterpret : xbsIndex_r4/Reinterpret  force_arith_type=off  arith_type=Unsigned  force_bin_pt=on  bin_pt=0  block_type=reinterpret
  Relational : xbsIndex_r4/Relational  mode=a>=b  en=off  latency=1  dbl_ovrd=off  block_type=relational
  sum_sumsq : Outport
  tag scope: adc_clip0=global
  wires:
  in/1 -> Reinterpret/1
  [adc_rms_rst] -> Accumulator/2, Accumulator1/2, Register/2, Register1/2
  Register/1 -> BitBasher/2
  Accumulator/1 -> Register/1
  Mult/1 -> Accumulator/1, Relational/1
  Register1/1 -> BitBasher/1
  Accumulator1/1 -> Register1/1
  Delay/1 -> Accumulator1/1
  BitBasher/1 -> sum_sumsq/1
  Delay1/1 -> Mult/2, Mult/1, Delay/1
  Reinterpret/1 -> Delay1/1
  Constant/1 -> Relational/2
  Relational/1 -> [adc_clip0]

== system roach2_fengine_nlb/input/rms/calc_adc_sum_sq1 ==
  note: 127^2 == 16129
  in : Inport
  Accumulator : xbsIndex_r4/Accumulator  operation=Add  n_bits=32  overflow=Wrap  scale=1  rst=on  infoeditControl=reset for floating point data type must be asserted for a minimum of 2 cycles  hasbypass=on  en=off  latency=0  dbl_ovrd=off  msb_inp=100  msb=100  lsb=-100  use_behavioral_HDL=on  implementation=Fabric  block_type=accum
      settings: infoedit="Adder or subtractor-based accumulator.   Output type and binary point position match the input.<P><P>Hardware notes: When \"Reinitialize with input 'b' on reset\" is selected, the accumulator is forced to run at the system rate even if the input 'b' is running at a slower rate."  xl_area=[0, 0, 0, 0, 0, 0, 0]  block_version=10.1.3
  Accumulator1 : xbsIndex_r4/Accumulator  operation=Add  n_bits=24  overflow=Wrap  scale=1  rst=on  infoeditControl=reset for floating point data type must be asserted for a minimum of 2 cycles  hasbypass=on  en=off  latency=0  dbl_ovrd=off  msb_inp=100  msb=100  lsb=-100  use_behavioral_HDL=on  implementation=Fabric  block_type=accum
      settings: infoedit="Adder or subtractor-based accumulator.   Output type and binary point position match the input.<P><P>Hardware notes: When \"Reinitialize with input 'b' on reset\" is selected, the accumulator is forced to run at the system rate even if the input 'b' is running at a slower rate."  xl_area=[0, 0, 0, 0, 0, 0, 0]  block_version=10.1.3
  BitBasher : xbsIndex_r4/BitBasher  bitexpr=|  display_expr=off  sr_1=1  arith_type1="Signed  (2's comp)"  bin_pt1=0  sr_2=2  arith_type2=Unsigned  bin_pt2=0  sr_3=3  arith_type3=Unsigned  bin_pt3=0  sr_4=4  arith_type4=Unsigned  bin_pt4=0  dbl_ovrd=off  block_type=bitbasher
      | <html><head><meta name="qrichtext" content="1" /><style type="text/css">
      | p, li { white-space: pre-wrap; }
      | </style></head><body style=" font-family:'MS Shell Dlg 2'; font-size:8.25pt; font-weight:400; font-style:normal;">
      | <p style=" margin-top:12px; margin-bottom:12px; margin-left:0px; margin-right:0px; -qt-block-indent:0; text-indent:0px; font-family:'MS Shell Dlg'; font-size:8pt;">sss={s,ss}</p></body></html>
      settings: block_version=10.1.3
  Constant : xbsIndex_r4/Constant  const=127^2  gui_display_data_type=Fixed-point  arith_type=Unsigned  n_bits=15  bin_pt=0  preci_type=Single  exp_width=8  frac_width=24  explicit_period=on  period=1  equ=P=C  opselect=C  inp2=PCIN>>17  opr=+  inp1=P  carry=CIN  dbl_ovrd=off  block_type=constant
  Delay : xbsIndex_r4/Delay  rst=off  infoeditControl=Selection of Reset will increase slice count due to use of real FFs and instead of SRLs  en=off  latency=2  dbl_ovrd=off  reg_retiming=off  block_type=delay
  Delay1 : xbsIndex_r4/Delay  rst=off  infoeditControl=Selection of Reset will increase slice count due to use of real FFs and instead of SRLs  en=off  latency=1  dbl_ovrd=off  reg_retiming=off  block_type=delay
  Mult : xbsIndex_r4/Mult  precision=User Defined  arith_type=Unsigned  n_bits=15  bin_pt=0  quantization=Truncate  overflow=Wrap  en=off  latency=2  dbl_ovrd=off  use_behavioral_HDL=on  opt=Speed  use_embedded=on  optimum_pipeline=on  pipeline=on  use_rpm=on  placement_style=Rectangular shape  block_type=mult
      settings: xl_area=[0, 0, 0, 0, 0, 0, 0]  block_version=10.1.3
  Register : xbsIndex_r4/Register  init=0  rst=off  en=on  dbl_ovrd=off  block_type=register
      settings: xl_area=[0, 0, 0, 0, 0, 0, 0]
  Register1 : xbsIndex_r4/Register  init=0  rst=off  en=on  dbl_ovrd=off  block_type=register
      settings: xl_area=[0, 0, 0, 0, 0, 0, 0]
  Reinterpret : xbsIndex_r4/Reinterpret  force_arith_type=off  arith_type=Unsigned  force_bin_pt=on  bin_pt=0  block_type=reinterpret
  Relational : xbsIndex_r4/Relational  mode=a>=b  en=off  latency=1  dbl_ovrd=off  block_type=relational
  sum_sumsq : Outport
  tag scope: adc_clip1=global
  wires:
  Relational/1 -> [adc_clip1]
  Constant/1 -> Relational/2
  Reinterpret/1 -> Delay1/1
  Delay1/1 -> Delay/1, Mult/1, Mult/2
  BitBasher/1 -> sum_sumsq/1
  Delay/1 -> Accumulator1/1
  Accumulator1/1 -> Register1/1
  Register1/1 -> BitBasher/1
  Mult/1 -> Relational/1, Accumulator/1
  Accumulator/1 -> Register/1
  Register/1 -> BitBasher/2
  [adc_rms_rst] -> Register1/2, Register/2, Accumulator1/2, Accumulator/2
  in/1 -> Reinterpret/1

== system roach2_fengine_nlb/input/rms/calc_adc_sum_sq10 ==
  note: 127^2 == 16129
  in : Inport
  Accumulator : xbsIndex_r4/Accumulator  operation=Add  n_bits=32  overflow=Wrap  scale=1  rst=on  infoeditControl=reset for floating point data type must be asserted for a minimum of 2 cycles  hasbypass=on  en=off  latency=0  dbl_ovrd=off  msb_inp=100  msb=100  lsb=-100  use_behavioral_HDL=on  implementation=Fabric  block_type=accum
      settings: infoedit="Adder or subtractor-based accumulator.   Output type and binary point position match the input.<P><P>Hardware notes: When \"Reinitialize with input 'b' on reset\" is selected, the accumulator is forced to run at the system rate even if the input 'b' is running at a slower rate."  xl_area=[0, 0, 0, 0, 0, 0, 0]  block_version=10.1.3
  Accumulator1 : xbsIndex_r4/Accumulator  operation=Add  n_bits=24  overflow=Wrap  scale=1  rst=on  infoeditControl=reset for floating point data type must be asserted for a minimum of 2 cycles  hasbypass=on  en=off  latency=0  dbl_ovrd=off  msb_inp=100  msb=100  lsb=-100  use_behavioral_HDL=on  implementation=Fabric  block_type=accum
      settings: infoedit="Adder or subtractor-based accumulator.   Output type and binary point position match the input.<P><P>Hardware notes: When \"Reinitialize with input 'b' on reset\" is selected, the accumulator is forced to run at the system rate even if the input 'b' is running at a slower rate."  xl_area=[0, 0, 0, 0, 0, 0, 0]  block_version=10.1.3
  BitBasher : xbsIndex_r4/BitBasher  bitexpr=|  display_expr=off  sr_1=1  arith_type1="Signed  (2's comp)"  bin_pt1=0  sr_2=2  arith_type2=Unsigned  bin_pt2=0  sr_3=3  arith_type3=Unsigned  bin_pt3=0  sr_4=4  arith_type4=Unsigned  bin_pt4=0  dbl_ovrd=off  block_type=bitbasher
      | <html><head><meta name="qrichtext" content="1" /><style type="text/css">
      | p, li { white-space: pre-wrap; }
      | </style></head><body style=" font-family:'MS Shell Dlg 2'; font-size:8.25pt; font-weight:400; font-style:normal;">
      | <p style=" margin-top:12px; margin-bottom:12px; margin-left:0px; margin-right:0px; -qt-block-indent:0; text-indent:0px; font-family:'MS Shell Dlg'; font-size:8pt;">sss={s,ss}</p></body></html>
      settings: block_version=10.1.3
  Constant : xbsIndex_r4/Constant  const=127^2  gui_display_data_type=Fixed-point  arith_type=Unsigned  n_bits=15  bin_pt=0  preci_type=Single  exp_width=8  frac_width=24  explicit_period=on  period=1  equ=P=C  opselect=C  inp2=PCIN>>17  opr=+  inp1=P  carry=CIN  dbl_ovrd=off  block_type=constant
  Delay : xbsIndex_r4/Delay  rst=off  infoeditControl=Selection of Reset will increase slice count due to use of real FFs and instead of SRLs  en=off  latency=2  dbl_ovrd=off  reg_retiming=off  block_type=delay
  Delay1 : xbsIndex_r4/Delay  rst=off  infoeditControl=Selection of Reset will increase slice count due to use of real FFs and instead of SRLs  en=off  latency=1  dbl_ovrd=off  reg_retiming=off  block_type=delay
  Mult : xbsIndex_r4/Mult  precision=User Defined  arith_type=Unsigned  n_bits=15  bin_pt=0  quantization=Truncate  overflow=Wrap  en=off  latency=2  dbl_ovrd=off  use_behavioral_HDL=on  opt=Speed  use_embedded=on  optimum_pipeline=on  pipeline=on  use_rpm=on  placement_style=Rectangular shape  block_type=mult
      settings: xl_area=[0, 0, 0, 0, 0, 0, 0]  block_version=10.1.3
  Register : xbsIndex_r4/Register  init=0  rst=off  en=on  dbl_ovrd=off  block_type=register
      settings: xl_area=[0, 0, 0, 0, 0, 0, 0]
  Register1 : xbsIndex_r4/Register  init=0  rst=off  en=on  dbl_ovrd=off  block_type=register
      settings: xl_area=[0, 0, 0, 0, 0, 0, 0]
  Reinterpret : xbsIndex_r4/Reinterpret  force_arith_type=off  arith_type=Unsigned  force_bin_pt=on  bin_pt=0  block_type=reinterpret
  Relational : xbsIndex_r4/Relational  mode=a>=b  en=off  latency=1  dbl_ovrd=off  block_type=relational
  sum_sumsq : Outport
  tag scope: adc_clip10=global
  wires:
  in/1 -> Reinterpret/1
  [adc_rms_rst] -> Accumulator/2, Accumulator1/2, Register/2, Register1/2
  Register/1 -> BitBasher/2
  Accumulator/1 -> Register/1
  Mult/1 -> Accumulator/1, Relational/1
  Register1/1 -> BitBasher/1
  Accumulator1/1 -> Register1/1
  Delay/1 -> Accumulator1/1
  BitBasher/1 -> sum_sumsq/1
  Delay1/1 -> Mult/2, Mult/1, Delay/1
  Reinterpret/1 -> Delay1/1
  Constant/1 -> Relational/2
  Relational/1 -> [adc_clip10]
